simulink model "Q2"  (R2021a)
settings: Solver=VariableStepAuto  StartTime=0.0  StopTime=10.0  RelTol=1e-3
libraries: simulink x1
settings Model: Creator=M.M  LastModifiedBy=M.M

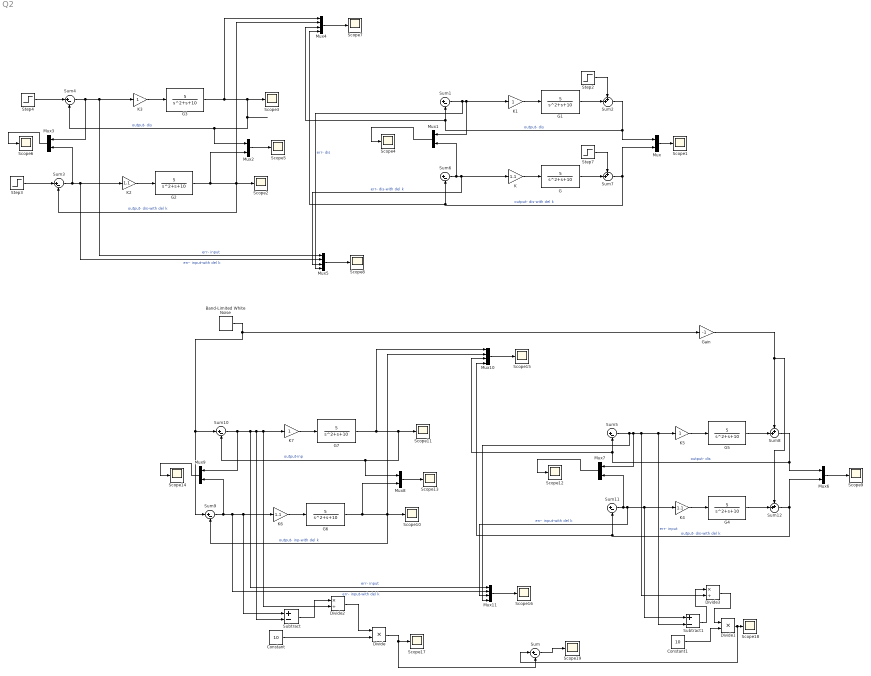
== system Q2 ==
  Band-Limited White Noise : simulink/Sources/Band-Limited White Noise  Cov=[1]  Ts=0.1  seed=[23341]
  Constant : Constant  Value=10
  Constant1 : Constant  Value=10
  Divide : Product  Inputs=**
  Divide1 : Product  Inputs=**
  Divide2 : Product  Inputs=*/
  Divide3 : Product  Inputs=*/
  G{,1..7} (8 alike) : TransferFcn  Numerator=[5]  Denominator=[1 1 10]
  Gain : Gain  Gain=-1
  K{,2,4,6} (4 alike) : Gain  Gain=1.1
  K{1,3,5,7} (4 alike) : Gain
  Mux{,1..3,6..9} (8 alike) : Mux  Inputs=2
  Mux{4..5,10..11} (4 alike) : Mux
  Scope{1..19} (19 alike) : Scope
  Step2 : Step  Time=0  After=-1  SampleTime=0
  Step3 : Step  Time=0  SampleTime=0
  Step4 : Step  Time=0  SampleTime=0
  Step7 : Step  Time=0  After=-1  SampleTime=0
  Subtract : Sum  Inputs=+-
  Subtract1 : Sum  Inputs=+-
  Sum{,1,3..6,9..11} (9 alike) : Sum  Inputs=|+-
  Sum{2,7..8,12} (4 alike) : Sum  Inputs=++|
  wires:
  Step7/1 -> Sum7/1
  Sum6/1 -> Mux1/2, Mux5/3, K/1  "err- dis-with del k"
  K/1 -> G/1
  Sum7/1 -> Mux/2, Mux4/4, Sum6/2  "output- dis-with del k"
  G/1 -> Sum7/2
  K1/1 -> G1/1
  Sum1/1 -> Mux5/4, Mux1/1, K1/1  "err- dis"
  G1/1 -> Sum2/2
  Sum2/1 -> Mux/1, Mux4/3, Sum1/2  "output- dis"
  Step2/1 -> Sum2/1
  K2/1 -> G2/1
  Sum3/1 -> Mux3/2, Mux5/2, K2/1  "err- input-with del k"
  Step3/1 -> Sum3/1
  K3/1 -> G3/1
  Sum4/1 -> Mux3/1, Mux5/1, K3/1  "err- input"
  Step4/1 -> Sum4/1
  Mux/1 -> Scope1/1
  Mux1/1 -> Scope4/1
  Mux2/1 -> Scope5/1
  G2/1 -> Mux2/2, Sum3/2, Mux4/2, Scope2/1  "output- dis-with del k"
  G3/1 -> Mux4/1, Scope3/1, Mux2/1, Sum4/2  "output- dis"
  Mux3/1 -> Scope6/1
  Mux4/1 -> Scope7/1
  Mux5/1 -> Scope8/1
  K6/1 -> G6/1
  Mux7/1 -> Scope12/1
  Mux11/1 -> Scope16/1
  Mux8/1 -> Scope13/1
  G7/1 -> Mux10/1, Scope11/1, Mux8/1, Sum10/2  "output-inp"
  Sum10/1 -> Mux9/1, Subtract/2, Divide2/2, K7/1, Mux11/1  "err- input"
  K7/1 -> G7/1
  G6/1 -> Mux8/2, Sum9/2, Mux10/2, Scope10/1  "output- inp-with del k"
  Mux9/1 -> Scope14/1
  Mux10/1 -> Scope15/1
  Sum9/1 -> Mux9/2, Mux11/2, Subtract/1, K6/1  "err- input-with del k"
  K4/1 -> G4/1
  Gain/1 -> Sum12/1, Sum8/1
  Mux6/1 -> Scope9/1
  Sum12/1 -> Mux6/2, Mux10/4, Sum11/2  "output- dis-with del k"
  G4/1 -> Sum12/2
  Sum8/1 -> Mux6/1, Mux10/3, Sum5/2  "output- dis"
  K5/1 -> G5/1
  G5/1 -> Sum8/2
  Band-Limited White Noise/1 -> Sum10/1, Sum9/1, Gain/1
  Constant/1 -> Divide/2
  Divide/1 -> Sum/2, Scope17/1
  Sum11/1 -> Mux7/2, Mux11/3, Subtract1/1, K4/1  "err- input-with del k"
  Divide1/1 -> Sum/1, Scope18/1
  Constant1/1 -> Divide1/2
  Sum5/1 -> Mux11/4, Mux7/1, Divide3/2, Subtract1/2, K5/1  "err- input"
  Subtract1/1 -> Divide3/1
  Subtract/1 -> Divide2/1
  Divide2/1 -> Divide/1
  Divide3/1 -> Divide1/1
  Sum/1 -> Scope19/1
